simulink library "Resettable_Integrator"  (R2020b)
settings: Solver=VariableStepAuto  StartTime=0.0  StopTime=10.0  RelTol=1e-3
undefined symbols (not defined in the file or in its folder): DiscIntNeverNeededParam, en_ResetStates, PauseResume
settings Model: Creator=matteolarcher  LastModifiedBy=matteolarcher

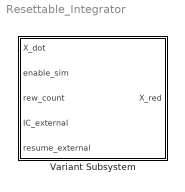
== system Resettable_Integrator ==
  Variant Subsystem : Subsystem  Variant=on  mask{Ts_int=1, L_up=inf, L_low=-inf, en_res_flag=en_ResetStates}
      mask prompts: Ts_int "sampling time"; L_up "upper saturation limit"; L_low "lower saturation limit"; en_res_flag "enable reset flag"

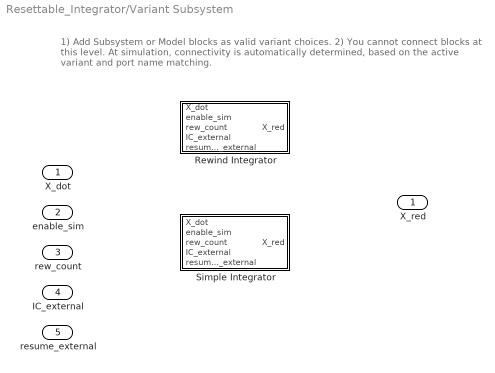
== system Resettable_Integrator/Variant Subsystem ==
  note: 1) Add Subsystem or Model blocks as valid variant choices.
      | 2) You cannot connect blocks at this level. At simulation, connectivity is automatically
      | determined, based on the active variant and port name matching.
  X_dot : Inport  OutDataTypeStr=double
  enable_sim : Inport  Port=2  OutDataTypeStr=boolean
  rew_count : Inport  Port=3  OutDataTypeStr=int16
  IC_external : Inport  Port=4  OutDataTypeStr=double
  resume_external : Inport  Port=5  OutDataTypeStr=double
  Rewind Integrator : Subsystem  VariantControl=en_res_flag == 1
  Simple Integrator : Subsystem  VariantControl=en_res_flag == 0
  X_red : Outport  OutDataTypeStr=double

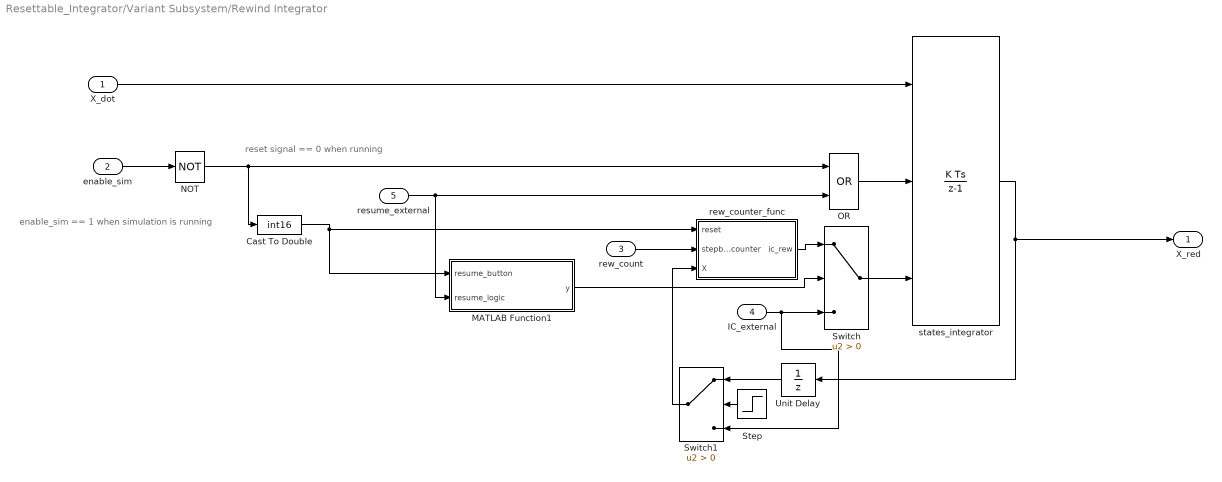
== system Resettable_Integrator/Variant Subsystem/Rewind Integrator ==
  note: reset signal == 0 when running
  note: enable_sim == 1 when simulation is running
  X_dot : Inport
  enable_sim : Inport  Port=2
  rew_count : Inport  Port=3
  IC_external : Inport  Port=4
  resume_external : Inport  Port=5
  Cast To Double : DataTypeConversion  OutDataTypeStr=int16
  MATLAB Function1 : MATLAB Function  TreatAsAtomicUnit=on
  NOT : Logic  Operator=NOT  IconShape=distinctive  AllPortsSameDT=off  OutDataTypeStr=boolean
  OR : Logic  Operator=OR  IconShape=distinctive  AllPortsSameDT=off  OutDataTypeStr=boolean
  Step : Step  Time=Ts_int
  Switch : Switch  Criteria=u2 > Threshold
  Switch1 : Switch  Criteria=u2 > Threshold
  Unit Delay : UnitDelay  SampleTime=-1  HasFrameUpgradeWarning=on
  rew_counter_func : MATLAB Function  TreatAsAtomicUnit=on
  states_integrator : DiscreteIntegrator  gainval=1  ExternalReset=level  InitialConditionSource=external  SampleTime=Ts_int  LimitOutput=on  UpperSaturationLimit=L_up  LowerSaturationLimit=L_low  ICPrevOutput=DiscIntNeverNeededParam  ICPrevScaledInput=DiscIntNeverNeededParam
  X_red : Outport
  wires:
  OR/1 -> states_integrator/2
  Switch1/1 -> rew_counter_func/3(X)
  rew_count/1 -> rew_counter_func/2(stepback_counter)
  enable_sim/1 -> NOT/1
  MATLAB Function1/1(y) -> Switch/2
  states_integrator/1 -> Unit Delay/1, X_red/1
  X_dot/1 -> states_integrator/1
  resume_external/1 -> MATLAB Function1/2(resume_logic), OR/2
  NOT/1 -> Cast To Double/1, OR/1
  Cast To Double/1 -> MATLAB Function1/1(resume_button), rew_counter_func/1(reset)
  Switch/1 -> states_integrator/3
  rew_counter_func/1(ic_rew) -> Switch/1
  Step/1 -> Switch1/2
  IC_external/1 -> Switch1/3, Switch/3
  Unit Delay/1 -> Switch1/1

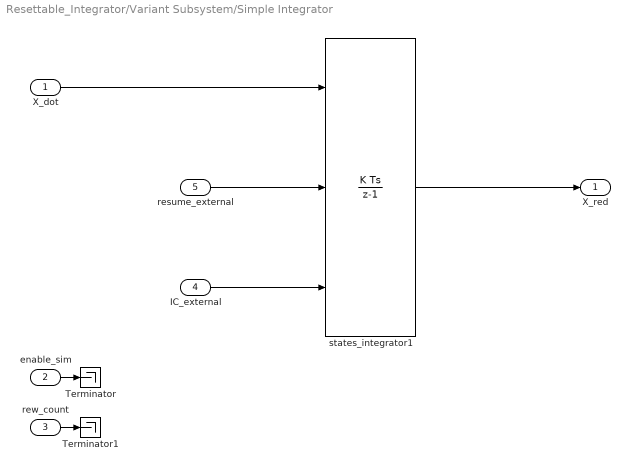
== system Resettable_Integrator/Variant Subsystem/Simple Integrator ==
  X_dot : Inport
  enable_sim : Inport  Port=2
  rew_count : Inport  Port=3
  IC_external : Inport  Port=4
  resume_external : Inport  Port=5
  Terminator : Terminator
  Terminator1 : Terminator
  states_integrator1 : DiscreteIntegrator  gainval=1  ExternalReset=rising  InitialConditionSource=external  SampleTime=Ts_int  LimitOutput=on  UpperSaturationLimit=L_up  LowerSaturationLimit=L_low  ICPrevOutput=DiscIntNeverNeededParam  ICPrevScaledInput=DiscIntNeverNeededParam
  X_red : Outport
  wires:
  X_dot/1 -> states_integrator1/1
  states_integrator1/1 -> X_red/1
  enable_sim/1 -> Terminator/1
  rew_count/1 -> Terminator1/1
  resume_external/1 -> states_integrator1/2
  IC_external/1 -> states_integrator1/3

== matlab function Resettable_Integrator/Variant Subsystem/Rewind Integrator/MATLAB Function1 ==
  data: resume_button input; y output; resume_logic input
function y = select_IC(resume_button, resume_logic)

tmp=1;

if (resume_button > 0 && resume_logic <= 0)
    tmp=1;
elseif (resume_button <= 0 && resume_logic > 0)
    tmp=-1;
elseif (resume_button > 0 && resume_logic >= 0)
    tmp=1;
end

y = tmp;

== matlab function Resettable_Integrator/Variant Subsystem/Rewind Integrator/rew_counter_func ==
  data: reset input; stepback_counter input; X input; ic_rew output; Ts_int parameter; PauseResume parameter
%% VEHICLE REWIND STATES

function ic_rew = ic_buffer(reset, stepback_counter, X, Ts_int, PauseResume)

persistent states_buf i reset_pre

% safety saturations
if PauseResume.rewind_time > 50
    n_states = 50;
else
    n_states = PauseResume.rewind_time;
end
if stepback_counter > n_states
    stepback_counter = int16(n_states);
end

% initialization

size_fifo = size(X(:),1);
ic_rew = zeros(1,size_fifo);
if isempty(states_buf)
    states_buf = zeros(int16(n_states), size_fifo);
    for j=1:n_states
        states_buf(j,:) = X;
    end
end
if isempty(i)
   i = 0;
end
if isempty(reset_pre)
   reset_pre = int16(0);
end

%%%%%%%%%%

% update buffer every rewind_samp 
if mod(i,PauseResume.rewind_samp/Ts_int)==0 && reset==0 && reset_pre==0
    states_buf(2:end,:) = states_buf(1:end-1,:);
    states_buf(1,:) = X;
end

% update initial conditions
if stepback_counter > 0     % stepback resume
    ic_rew(1,:) = states_buf(stepback_counter, :);
else                        % pause-resume without stepback 
    ic_rew(1,:) = X;
end

% detect enable falling edge and update buffer
% selected
if reset_pre > reset
    remain_size = n_states-stepback_counter+1;              % number of samples older than stepback_counter to be keep
    states_buf(1:remain_size, :) = states_buf(stepback_counter:end, :);    % porto in cima alla fifo i valori rimasti del buffer più vecchi di stepback_counter
    for j=remain_size+1:n_states
        states_buf(j, :) = states_buf(remain_size, :);         % riempio la fifo con l'ultimo valore buono 
    end
end

% increase counter
i = i+1;
reset_pre = reset;
     
end
